simulink model "Validation_Kalman_OP"  (R2019a)
settings: Solver=FixedStepAuto  StartTime=0.0  StopTime=100  FixedStep=sampleTime  RelTol=1e-3
values from neighbouring files (symbols this model uses):
  Kalman_OP = Setup_Kalman_OP(Q, R)    [Replay_Script.m]
  sampleTime = 0.05    [Replay_Script.m]
libraries: simulink x3
settings Model: Creator=Gaming  LastModifiedBy=User

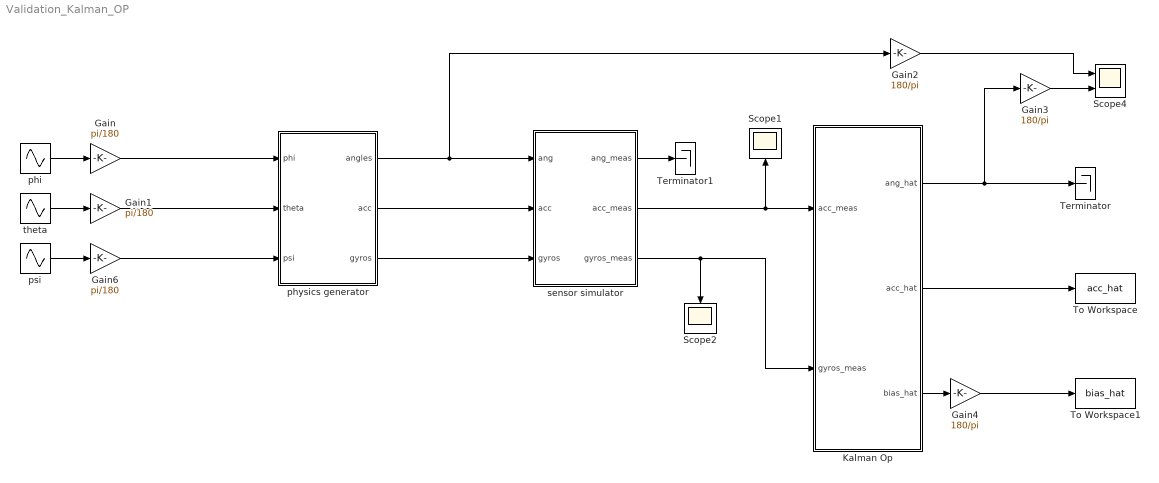
== system Validation_Kalman_OP ==
  Gain : Gain  Gain=pi/180
  Gain1 : Gain  Gain=pi/180
  Gain2 : Gain  Gain=180/pi
  Gain3 : Gain  Gain=180/pi
  Gain4 : Gain  Gain=180/pi
  Gain6 : Gain  Gain=pi/180
  Kalman Op : Subsystem
  Scope1 : Scope
  Scope2 : Scope
  Scope4 : Scope  NumInputPorts=2
  Terminator : Terminator
  Terminator1 : Terminator
  To Workspace : ToWorkspace  VariableName=acc_hat  SaveFormat=Structure With Time  SampleTime=-1
  To Workspace1 : ToWorkspace  VariableName=bias_hat  SaveFormat=Structure With Time  SampleTime=-1
  phi : Sin  Amplitude=12  Bias=6  Frequency=2*pi/10  SampleTime=0
  physics generator : Subsystem
  psi : Sin  Amplitude=0  Bias=10  Frequency=2*pi/5  Phase=pi  SampleTime=0
  sensor simulator : Subsystem
  theta : Sin  Amplitude=15  Frequency=2*pi/5  Phase=pi  SampleTime=0
  wires:
  phi/1 -> Gain/1
  theta/1 -> Gain1/1
  Kalman Op/3(bias_hat) -> Gain4/1
  Kalman Op/2(acc_hat) -> To Workspace/1
  Kalman Op/1(ang_hat) -> Terminator/1, Gain3/1
  Gain2/1 -> Scope4/1
  Gain3/1 -> Scope4/2
  Gain4/1 -> To Workspace1/1
  psi/1 -> Gain6/1
  Gain/1 -> physics generator/1(phi)
  Gain1/1 -> physics generator/2(theta)
  Gain6/1 -> physics generator/3(psi)
  physics generator/1(angles) -> Gain2/1, sensor simulator/1(ang)
  sensor simulator/2(acc_meas) -> Scope1/1, Kalman Op/1(acc_meas)
  sensor simulator/3(gyros_meas) -> Kalman Op/2(gyros_meas), Scope2/1
  physics generator/2(acc) -> sensor simulator/2(acc)
  physics generator/3(gyros) -> sensor simulator/3(gyros)
  sensor simulator/1(ang_meas) -> Terminator1/1

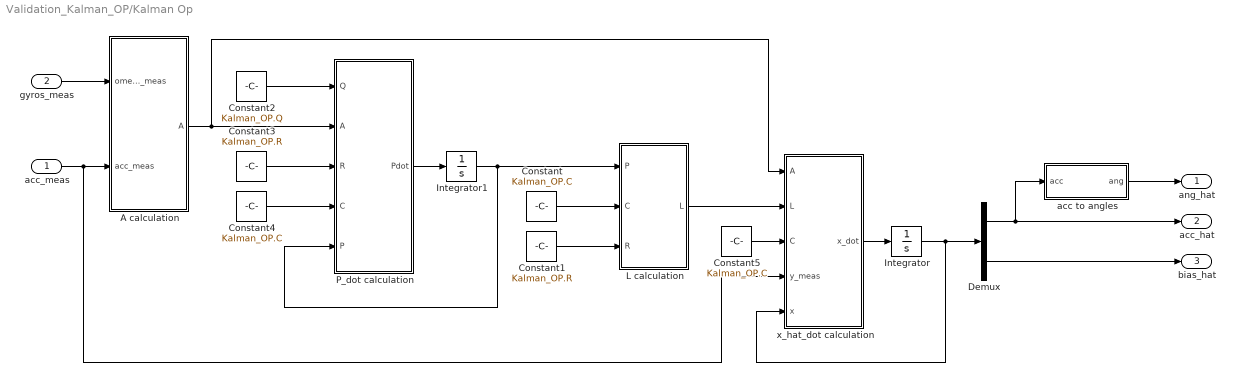
== system Validation_Kalman_OP/Kalman Op ==
  acc_meas : Inport
  gyros_meas : Inport  Port=2
  A calculation : MATLAB Function  TreatAsAtomicUnit=on
  Constant : Constant  Value=Kalman_OP.C
  Constant1 : Constant  Value=Kalman_OP.R
  Constant2 : Constant  Value=Kalman_OP.Q
  Constant3 : Constant  Value=Kalman_OP.R
  Constant4 : Constant  Value=Kalman_OP.C
  Constant5 : Constant  Value=Kalman_OP.C
  Demux : Demux  Outputs=2
  Integrator : Integrator  InitialCondition=zeros(6,1)
  Integrator1 : Integrator  InitialCondition=Kalman_OP.Q*10
  L calculation : MATLAB Function  TreatAsAtomicUnit=on
  P_dot calculation : MATLAB Function  TreatAsAtomicUnit=on
  acc to angles : MATLAB Function  TreatAsAtomicUnit=on
  x_hat_dot calculation : MATLAB Function  TreatAsAtomicUnit=on
  ang_hat : Outport
  acc_hat : Outport  Port=2
  bias_hat : Outport  Port=3
  wires:
  acc to angles/1(ang) -> ang_hat/1
  x_hat_dot calculation/1(x_dot) -> Integrator/1
  Integrator/1 -> Demux/1, x_hat_dot calculation/5(x)
  L calculation/1(L) -> x_hat_dot calculation/2(L)
  P_dot calculation/1(Pdot) -> Integrator1/1
  Integrator1/1 -> P_dot calculation/5(P), L calculation/1(P)
  Constant/1 -> L calculation/2(C)
  Constant1/1 -> L calculation/3(R)
  Constant3/1 -> P_dot calculation/3(R)
  Constant2/1 -> P_dot calculation/1(Q)
  Demux/1 -> acc to angles/1(acc), acc_hat/1
  Demux/2 -> bias_hat/1
  acc_meas/1 -> x_hat_dot calculation/4(y_meas), A calculation/2(acc_meas)
  gyros_meas/1 -> A calculation/1(omega_meas)
  A calculation/1(A) -> x_hat_dot calculation/1(A), P_dot calculation/2(A)
  Constant4/1 -> P_dot calculation/4(C)
  Constant5/1 -> x_hat_dot calculation/3(C)

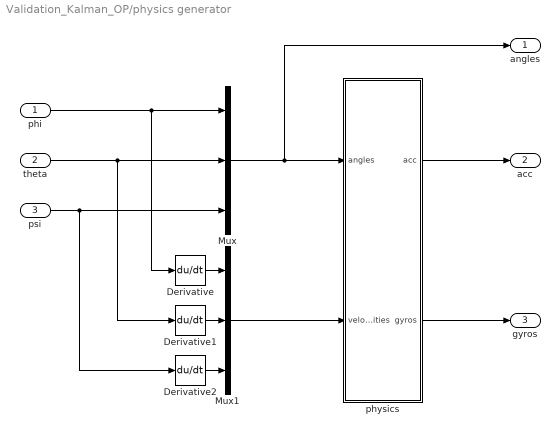
== system Validation_Kalman_OP/physics generator ==
  phi : Inport
  theta : Inport  Port=2
  psi : Inport  Port=3
  Derivative : Derivative
  Derivative1 : Derivative
  Derivative2 : Derivative
  Mux : Mux  Inputs=3
  Mux1 : Mux  Inputs=3
  physics : MATLAB Function  TreatAsAtomicUnit=on
  angles : Outport
  acc : Outport  Port=2
  gyros : Outport  Port=3
  wires:
  phi/1 -> Derivative/1, Mux/1
  Derivative2/1 -> Mux1/3
  psi/1 -> Derivative2/1, Mux/3
  physics/1(acc) -> acc/1
  theta/1 -> Derivative1/1, Mux/2
  Mux/1 -> angles/1, physics/1(angles)
  Derivative1/1 -> Mux1/2
  Derivative/1 -> Mux1/1
  Mux1/1 -> physics/2(velocities)
  physics/2(gyros) -> gyros/1

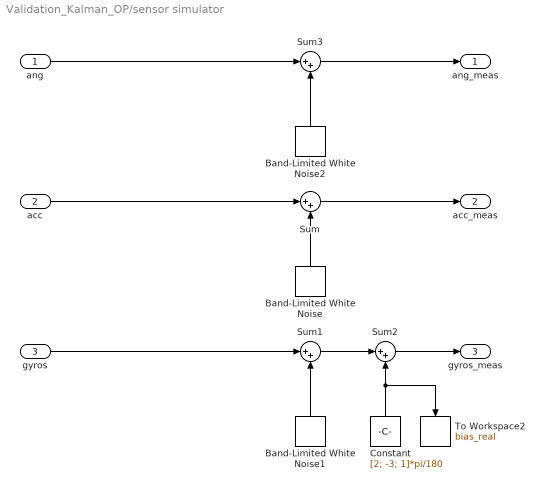
== system Validation_Kalman_OP/sensor simulator ==
  ang : Inport
  acc : Inport  Port=2
  gyros : Inport  Port=3
  Band-Limited White Noise : simulink/Sources/Band-Limited White Noise  Cov=[0.05^2*sampleTime]  Ts=sampleTime  seed=[23331]
  Band-Limited White Noise1 : simulink/Sources/Band-Limited White Noise  Cov=[(0.05*pi/180)^2*sampleTime]  Ts=sampleTime  seed=[23341]
  Band-Limited White Noise2 : simulink/Sources/Band-Limited White Noise  Cov=[0.05^2*sampleTime]  Ts=sampleTime  seed=[23331]
  Constant : Constant  Value=[2; -3; 1]*pi/180  VectorParams1D=off
  Sum{,1..3} (4 alike) : Sum  Inputs=|++
  To Workspace2 : ToWorkspace  VariableName=bias_real  SaveFormat=Structure With Time  SampleTime=-1
  ang_meas : Outport
  acc_meas : Outport  Port=2
  gyros_meas : Outport  Port=3
  wires:
  acc/1 -> Sum/1
  Band-Limited White Noise/1 -> Sum/2
  Constant/1 -> To Workspace2/1, Sum2/2
  Sum2/1 -> gyros_meas/1
  Sum1/1 -> Sum2/1
  Sum/1 -> acc_meas/1
  Band-Limited White Noise1/1 -> Sum1/2
  gyros/1 -> Sum1/1
  Sum3/1 -> ang_meas/1
  ang/1 -> Sum3/1
  Band-Limited White Noise2/1 -> Sum3/2

== matlab function Validation_Kalman_OP/Kalman Op/P_dot calculation ==
  data: Q input; A input; Pdot output; R input; C input; P input
function Pdot = fcn(Q, A, R, C, P)

Pdot = A*P + P*transpose(A) + Q - P*transpose(C)*inv(R)*C*P;

== matlab function Validation_Kalman_OP/physics generator/physics ==
  data: angles input; acc output; velocities input; gyros output
function [acc,gyros] = fcn(angles, velocities)

% angles - phi, theta

acc = -10*[-sin(angles(2)); cos(angles(2))*sin(angles(1));cos(angles(2))*cos(angles(1))];

A = [1, sin(velocities(1))*tan(velocities(2))   , cos(velocities(1))*tan(velocities(2)) ;...
     0, cos(velocities(1))                      , -sin(velocities(1))                   ;...
     0, sin(velocities(1))/cos(velocities(2))   , cos(velocities(1))/cos(velocities(2))];


gyros = A\[velocities];

== matlab function Validation_Kalman_OP/Kalman Op/acc to angles ==
  data: acc input; ang output
function ang = fcn(acc)

phi = -atan2(acc(2),-acc(3));

theta = atan2(acc(1),sqrt(acc(2)^2+acc(3)^2));

ang = [phi; theta];

== matlab function Validation_Kalman_OP/Kalman Op/L calculation ==
  data: P input; L output; C input; R input
function L = fcn(P, C, R)

L = P*transpose(C)*inv(R);

== matlab function Validation_Kalman_OP/Kalman Op/x_hat_dot calculation ==
  data: A input; x_dot output; L input; C input; y_meas input; x input
function x_dot = fcn(A,L,C,y_meas,x)

x_dot = A*x + L*(y_meas - C*x);

== matlab function Validation_Kalman_OP/Kalman Op/A calculation ==
  data: omega_meas input; A output; acc_meas input
function A = fcn(omega_meas, acc_meas)

w = omega_meas;
a = acc_meas;

s_1 = [ 0   , -w(3) ,  w(2) ;...
        w(3),  0    , -w(1) ;...
       -w(2),  w(1) ,  0    ];
   
s_2 = [ 0   , -a(3) ,  a(2) ;...
        a(3),  0    , -a(1) ;...
       -a(2),  a(1) ,  0    ];
   
A = [-s_1, -s_2 ;...
     zeros(3,6) ];
